simulink subsystem "dq_dt"  (R2020b)
settings: Solver=VariableStepAuto  StartTime=0.0  StopTime=10.0  RelTol=1e-3
settings Model: Creator=newpo  LastModifiedBy=newpo

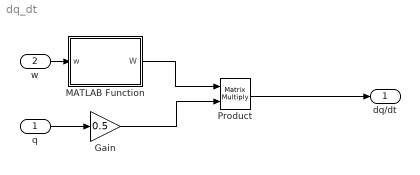
== system dq_dt ==
  q : Inport
  w : Inport  Port=2
  Gain : Gain  Gain=0.5
  MATLAB Function : MATLAB Function  TreatAsAtomicUnit=on
  Product : Product  Multiplication=Matrix(*)
  dq/dt : Outport
  wires:
  w/1 -> MATLAB Function/1(w)
  q/1 -> Gain/1
  MATLAB Function/1(W) -> Product/1
  Gain/1 -> Product/2
  Product/1 -> dq/dt/1

== matlab function dq_dt/MATLAB Function ==
  data: w input; W output
function W = make_Omega(w)
    W = [   0     w(3)  -w(2)  w(1); 
           -w(3)  0     w(1)   w(2);
            w(2) -w(1)   0     w(3);
           -w(1) -w(2)  -w(3)  0    ] ; 
end
